simulink model "out_put"  (R2019b)
settings: Solver=ode1  StartTime=ts  StopTime=10.0  FixedStep=dt  RelTol=1e-3
(part 3 of 3)

== system out_put/input_euler_angle_roll_pitch_euler_rate_yaw2/__InputSSForSFun__ ==

== system out_put/input_euler_angle_roll_pitch_euler_rate_yaw2/__OutputSSForSFun__ ==
